simulink model "Simulacao_2B"  (R2015a)
settings: Solver=ode45  StartTime=0.0  StopTime=240  FixedStep=0.1  MaxStep=5e-1  RelTol=1e-3
libraries: simulink x6
settings Model: CovSFcnEnable=off  Creator=MeneghettiAir  LastModifiedBy=hemerson
settings DebuggingCC: SolverPrmCheckMsg=warning

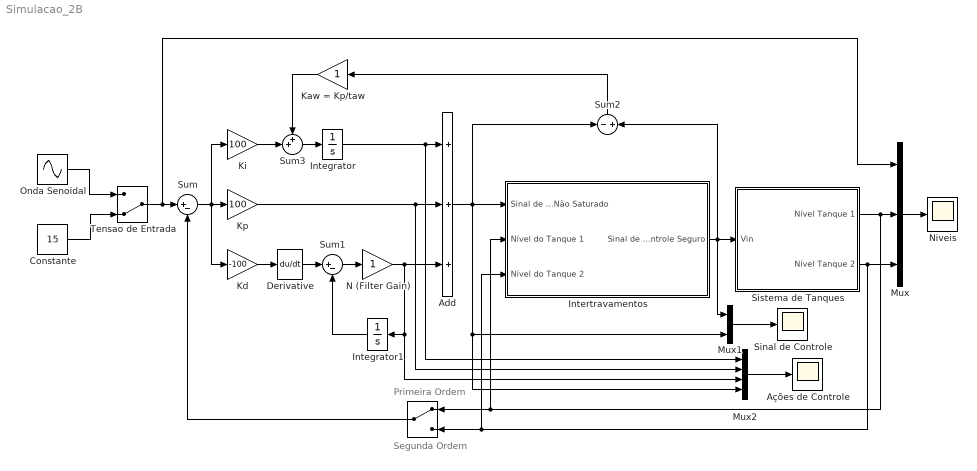
== system Simulacao_2B ==
  note: Segunda Ordem
  note: Primeira Ordem
  "\tAções de Controle" : Scope
      settings: ShowLegends=on  TimeRange=240  MaxDataPoints=500000
  " " : ManualSwitch
  Add : Sum  Inputs=+++
  Constante : Constant  Value=15
  Derivative : Derivative
  Integrator : Integrator
  Integrator1 : Integrator
  Intertravamentos : Subsystem
  Kaw = Kp/taw : Gain
  Kd : Gain  Gain=-100
  Ki : Gain  Gain=100
  Kp : Gain  Gain=100
  Mux : Mux  Inputs=3
  Mux1 : Mux  Inputs=2
  Mux2 : Mux
  N (Filter Gain) : Gain
  Niveis : Scope
      settings: ShowLegends=on  TimeRange=240  YMax=35  SaveName=Niveis  MaxDataPoints=500000
  Onda Senoidal : Sin  Amplitude=2  Bias=2  Frequency=0.2  SampleTime=0
  Sinal de Controle : Scope
      settings: ShowLegends=on  TimeRange=240  YMin=-1  YMax=6  MaxDataPoints=500000
  "Sistema de Tanques " : Subsystem
  Sum : Sum  Inputs=|+-
  Sum1 : Sum  Inputs=|+-
  Sum2 : Sum  Inputs=-|+
  Sum3 : Sum  Inputs=++|
  Tensao de Entrada : ManualSwitch  CurrentSetting=0
  wires:
  "Sistema de Tanques "/2(Nível Tanque 2) -> " "/2, Intertravamentos/3(Nível do Tanque 2), Mux/3
  Mux/1 -> Niveis/1
  Constante/1 -> Tensao de Entrada/2
  Onda Senoidal/1 -> Tensao de Entrada/1
  Add/1 -> Intertravamentos/1(Sinal de Controle Não Saturado), Sum2/1, Mux2/4, Mux1/2
  Tensao de Entrada/1 -> Mux/1, Sum/1
  Mux1/1 -> Sinal de Controle/1
  Mux2/1 -> "\tAções de Controle"/1
  Sum/1 -> Kd/1, Kp/1, Ki/1
  Integrator/1 -> Mux2/1, Add/1
  Kd/1 -> Derivative/1
  Kp/1 -> Mux2/2, Add/2
  "Sistema de Tanques "/1(Nível Tanque 1) -> Mux/2, " "/1, Intertravamentos/2(Nível do Tanque 1)
  Derivative/1 -> Sum1/1
  Sum1/1 -> N (Filter Gain)/1
  N (Filter Gain)/1 -> Mux2/3, Integrator1/1, Add/3
  Integrator1/1 -> Sum1/2
  Ki/1 -> Sum3/2
  Sum3/1 -> Integrator/1
  Sum2/1 -> Kaw = Kp/taw/1
  Kaw = Kp/taw/1 -> Sum3/1
  Intertravamentos/1(Sinal de Controle Seguro) -> Sum2/2, "Sistema de Tanques "/1(Vin), Mux1/1
  " "/1 -> Sum/2

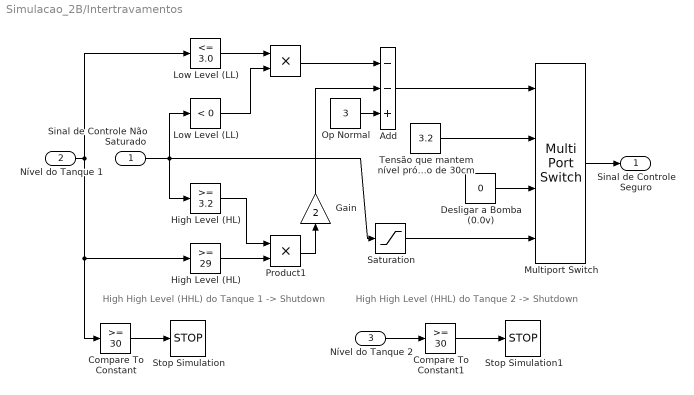
== system Simulacao_2B/Intertravamentos ==
  note: High High Level (HHL) do Tanque 1 -> Shutdown
  note: High High Level (HHL) do Tanque 2 -> Shutdown
  Sinal de Controle Não Saturado : Inport
  Nível do Tanque 1 : Inport  Port=2
  Nível do Tanque 2 : Inport  Port=3
  " " : Product
  " High Level (HL)" : simulink/Logic and Bit Operations/Compare To Constant  relop=>=  const=29  OutDataTypeStr=boolean
  " Low Level (LL) " : simulink/Logic and Bit Operations/Compare To Zero  relop=<  OutDataTypeStr=boolean
  Add : Sum  Inputs=--+
  Compare To Constant : simulink/Logic and Bit Operations/Compare To Constant  relop=>=  const=30  OutDataTypeStr=boolean
  Compare To Constant1 : simulink/Logic and Bit Operations/Compare To Constant  relop=>=  const=30  OutDataTypeStr=boolean
  Desligar a Bomba (0.0v) : Constant  Value=0
  Gain : Gain  Gain=2
  High Level (HL) : simulink/Logic and Bit Operations/Compare To Constant  relop=>=  const=3.2  OutDataTypeStr=boolean
  Low Level (LL) : simulink/Logic and Bit Operations/Compare To Constant  relop=<=  const=3.0  OutDataTypeStr=boolean
  Multiport Switch : MultiPortSwitch
  Op Normal : Constant  Value=3
  Product1 : Product
  Saturation : Saturate
  Stop Simulation : Stop
  Stop Simulation1 : Stop
  Tensão que mantem nível próximo de 30cm : Constant  Value=3.2
  Sinal de Controle Seguro : Outport
  wires:
  Compare To Constant1/1 -> Stop Simulation1/1
  Nível do Tanque 2/1 -> Compare To Constant1/1
  Compare To Constant/1 -> Stop Simulation/1
  Nível do Tanque 1/1 -> Low Level (LL)/1, " High Level (HL)"/1, Compare To Constant/1
  Desligar a Bomba (0.0v)/1 -> Multiport Switch/3
  Tensão que mantem nível próximo de 30cm/1 -> Multiport Switch/2
  Add/1 -> Multiport Switch/1
  Op Normal/1 -> Add/3
  Gain/1 -> Add/2
  Product1/1 -> Gain/1
  " "/1 -> Add/1
  Saturation/1 -> Multiport Switch/4
  " Low Level (LL) "/1 -> " "/2
  Low Level (LL)/1 -> " "/1
  High Level (HL)/1 -> Product1/1
  " High Level (HL)"/1 -> Product1/2
  Sinal de Controle Não Saturado/1 -> High Level (HL)/1, Saturation/1, " Low Level (LL) "/1
  Multiport Switch/1 -> Sinal de Controle Seguro/1

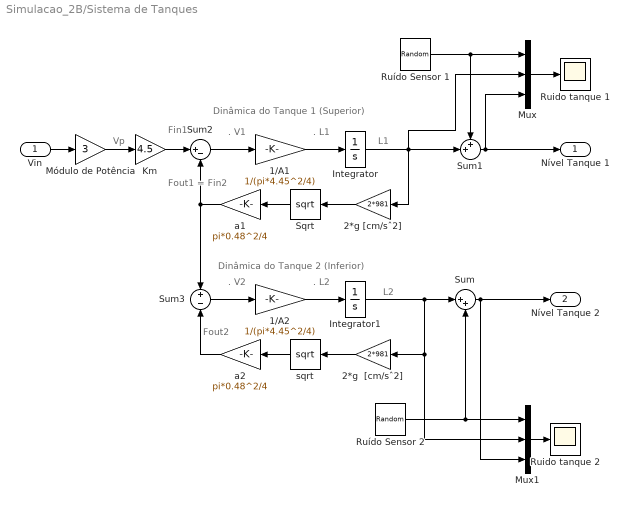
== system Simulacao_2B/Sistema de Tanques  ==
  note: Dinâmica do Tanque 1 (Superior)
  note: L1
  note: Fin1
  note: Fout1
      | =
      | Fin2
  note: .
      | L1
  note: .
      | V1
  note: L2
  note: Fout2
  note: .
      | L2
  note: .
      | V2
  note: Dinâmica do Tanque 2 (Inferior)
  note: Vp
  Vin : Inport
  1/A1 : Gain  Gain=1/(pi*4.45^2/4)
  1/A2 : Gain  Gain=1/(pi*4.45^2/4)
  2*g  [cm/sˆ2] : Gain  Gain=2*981
  2*g [cm/sˆ2] : Gain  Gain=2*981
  Integrator : Integrator  UpperSaturationLimit=35  LowerSaturationLimit=-2
  Integrator1 : Integrator  UpperSaturationLimit=35  LowerSaturationLimit=-2
  Km : Gain  Gain=4.5
  Mux : Mux  Inputs=3
  Mux1 : Mux  Inputs=3
  Módulo de Potência : Gain  Gain=3
  Ruido tanque 1 : Scope
      settings: TimeRange=50  YMin=0  YMax=20  SaveName=ScopeData3
  Ruido tanque 2 : Scope
      settings: TimeRange=50  YMin=0  YMax=20  SaveName=ScopeData4
  Ruído Sensor 1 : UniformRandomNumber  Minimum=-0.1  Maximum=0.1  Seed=round(rand(1)*100)  SampleTime=0.5
  Ruído Sensor 2 : UniformRandomNumber  Minimum=-0.1  Maximum=0.1  Seed=round(rand(1)*100)  SampleTime=0.7
  Sqrt : Sqrt  SaturateOnIntegerOverflow=on
  Sum : Sum  Inputs=|++
  Sum1 : Sum  Inputs=++|
  Sum2 : Sum  Inputs=|+-
  Sum3 : Sum  Inputs=+-
  a1 : Gain  Gain=pi*0.48^2/4
  a2 : Gain  Gain=pi*0.48^2/4
  sqrt : Sqrt  SaturateOnIntegerOverflow=on
  Nível Tanque 1 : Outport
  Nível Tanque 2 : Outport  Port=2
  wires:
  Vin/1 -> Módulo de Potência/1
  Sum/1 -> Nível Tanque 2/1, Mux1/3
  Mux/1 -> Ruido tanque 1/1
  Mux1/1 -> Ruido tanque 2/1
  Sum1/1 -> Nível Tanque 1/1, Mux/3
  Ruído Sensor 1/1 -> Mux/1, Sum1/1
  Ruído Sensor 2/1 -> Sum/2, Mux1/1
  2*g [cm/sˆ2]/1 -> Sqrt/1
  Sqrt/1 -> a1/1
  Km/1 -> Sum2/1
  a1/1 -> Sum2/2, Sum3/1
  Sum2/1 -> 1/A1/1
  1/A1/1 -> Integrator/1
  2*g  [cm/sˆ2]/1 -> sqrt/1
  sqrt/1 -> a2/1
  Sum3/1 -> 1/A2/1
  1/A2/1 -> Integrator1/1
  a2/1 -> Sum3/2
  Módulo de Potência/1 -> Km/1
  Integrator/1 -> Sum1/2, Mux/2, 2*g [cm/sˆ2]/1
  Integrator1/1 -> Mux1/2, 2*g  [cm/sˆ2]/1, Sum/1
